simulink model "ysw5_17"  (R2014a)
settings: Solver=ode45  StartTime=0.0  StopTime=10.0  RelTol=1e-3
settings Model: Creator=Administrator  LastModifiedBy=Administrator

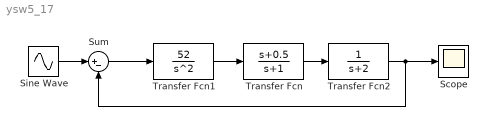
== system ysw5_17 ==
  Scope : Scope
  Sine Wave : Sin  SampleTime=0
  Sum : Sum  Inputs=|+-
  Transfer Fcn : TransferFcn  Numerator=[1 0.5]  Denominator=[1 1]
  Transfer Fcn1 : TransferFcn  Numerator=[52]  Denominator=[1 0 0]
  Transfer Fcn2 : TransferFcn  Numerator=1  Denominator=[1 2]
  wires:
  Sine Wave/1 -> Sum/1
  Transfer Fcn2/1 -> Sum/2, Scope/1
  Sum/1 -> Transfer Fcn1/1
  Transfer Fcn1/1 -> Transfer Fcn/1
  Transfer Fcn/1 -> Transfer Fcn2/1
